simulink model "fuzzysliding"  (R2020a)
settings: Solver=FixedStepAuto  StartTime=0.0  StopTime=10  FixedStep=Ts  RelTol=1e-3
values from neighbouring files (symbols this model uses):
  A_c = [0 1;0 0]    [fuzzysliding.m]    (also in fuzzytest.m)
  B_c = [0;Kx]    [fuzzysliding.m]    (also in fuzzytest.m = [0;K])
  C_c = [1 0]    [fuzzysliding.m]    (also in fuzzytest.m)
  D_c = 0    [fuzzysliding.m]    (also in fuzzytest.m)
  Kx = 5*g/7    (= 7.00714285714)    [fuzzysliding.m]
  lambdax = 1    [fuzzysliding.m]
  Ts = 0.02    [fuzzysliding.m]    (also in fuzzytest.m = 0.2)
libraries: simulink x4, fuzblock x1
settings Model: Creator=Ashraf  LastModifiedBy=hhiastt
settings DataIOCC: ReturnWorkspaceOutputs=off
settings DebuggingCC: ArithmeticOperatorsInVariantConditions=warning
settings SFSimCC: SimUseLocalCustomCode=off  CustomCodeUndefinedFunction=UseInterfaceOnly
settings RTWCC: RTWUseLocalCustomCode=off
settings CodeAppCC: StateflowObjectComments=on

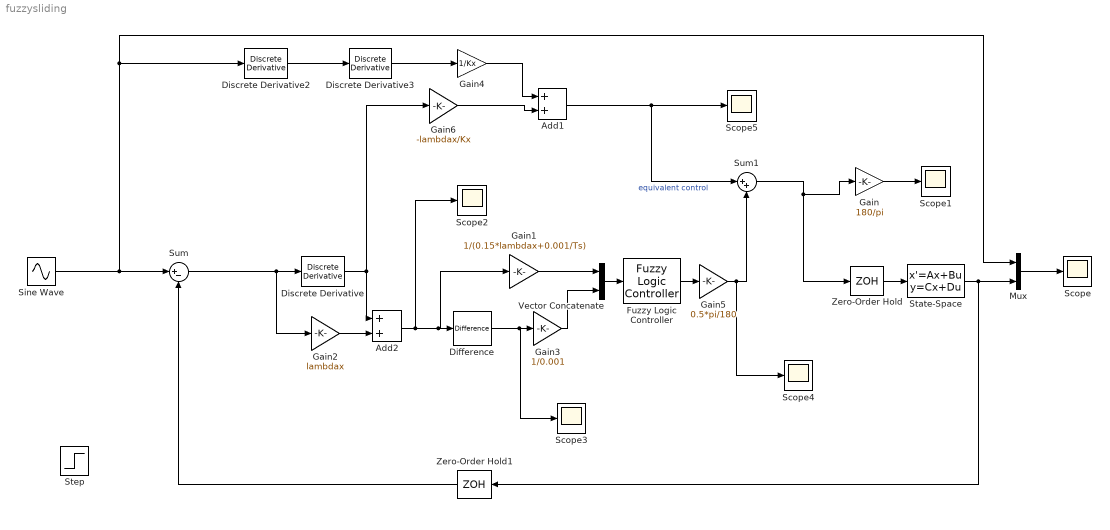
== system fuzzysliding ==
  Add1 : Sum
  Add2 : Sum
  Difference : simulink/Discrete/Difference  ICPrevInput=0.0  OutMin=[]  OutMax=[]  OutDataType=fixdt(1, 16)  OutScaling=2^-10  DoSatur=off
  Discrete Derivative : simulink/Discrete/Discrete Derivative  gainval=1.0  ICPrevScaledInput=0.0  OutMin=[]  OutMax=[]  OutDataType=fixdt(1, 16)  OutScaling=2^-10  DoSatur=off
  Discrete Derivative2 : simulink/Discrete/Discrete Derivative  gainval=1.0  ICPrevScaledInput=0.0  OutMin=[]  OutMax=[]  OutDataType=fixdt(1, 16)  OutScaling=2^-10  DoSatur=off
  Discrete Derivative3 : simulink/Discrete/Discrete Derivative  gainval=1.0  ICPrevScaledInput=0.0  OutMin=[]  OutMax=[]  OutDataType=fixdt(1, 16)  OutScaling=2^-10  DoSatur=off
  Fuzzy Logic Controller : fuzblock/Fuzzy Logic  Controller  FIS='fuzzysliding.fis'  OutputSampleNumber=101  DataType=double  FuzzifiedInputs=off  RuleFiringStrengths=off  RuleOutputs=off  AggregatedOutputs=off  SimulateUsing=Interpreted execution  OutOfRangeInputValueMessage=warning  NoRuleFiredMessage=warning  EmptyOutputFuzzySetMessage=warning
  Gain : Gain  Gain=180/pi
  Gain1 : Gain  Gain=1/(0.15*lambdax+0.001/Ts)
  Gain2 : Gain  Gain=lambdax
  Gain3 : Gain  Gain=1/0.001
  Gain4 : Gain  Gain=1/Kx
  Gain5 : Gain  Gain=0.5*pi/180
  Gain6 : Gain  Gain=-lambdax/Kx
  Mux : Mux  Inputs=2
  Scope{,1..5} (6 alike) : Scope
  Sine Wave : Sin  Amplitude=0.1  SampleTime=Ts
  State-Space : StateSpace  A=A_c  B=B_c  C=C_c  D=D_c  InitialCondition=0
  Step : Step  Time=0  After=0.1  SampleTime=Ts
  Sum : Sum  Inputs=|+-
  Sum1 : Sum  Inputs=|++
  Vector Concatenate : Concatenate
  Zero-Order Hold : ZeroOrderHold  SampleTime=Ts
  Zero-Order Hold1 : ZeroOrderHold  SampleTime=Ts
  wires:
  Zero-Order Hold/1 -> State-Space/1
  Fuzzy Logic Controller/1 -> Gain5/1
  State-Space/1 -> Zero-Order Hold1/1, Mux/2
  Vector Concatenate/1 -> Fuzzy Logic Controller/1
  Zero-Order Hold1/1 -> Sum/2
  Mux/1 -> Scope/1
  Sum/1 -> Gain2/1, Discrete Derivative/1
  Gain2/1 -> Add2/2
  Add2/1 -> Scope2/1, Gain1/1, Difference/1
  Gain1/1 -> Vector Concatenate/1
  Gain3/1 -> Vector Concatenate/2
  Difference/1 -> Scope3/1, Gain3/1
  Gain5/1 -> Scope4/1, Sum1/2
  Discrete Derivative3/1 -> Gain4/1
  Gain4/1 -> Add1/1
  Gain6/1 -> Add1/2
  Discrete Derivative/1 -> Add2/1, Gain6/1
  Discrete Derivative2/1 -> Discrete Derivative3/1
  Add1/1 -> Scope5/1, Sum1/1  "equivalent control"
  Sine Wave/1 -> Discrete Derivative2/1, Mux/1, Sum/1
  Gain/1 -> Scope1/1
  Sum1/1 -> Zero-Order Hold/1, Gain/1
